simulink model "twoControllers"  (R2019b)
settings: Solver=VariableStepAuto  StartTime=0.0  StopTime=10.0  RelTol=1e-3
values from neighbouring files (symbols this model uses):
  g = 9.81    [G.m]    (also in connect_pend_runner.m = -9.81; run.m; single_pend_runner.m = -9.81)
  Kd = 50    [anujay_single_pendulum_same.m]    (also in connect_pend_runner.m = 10; double_pend_setup.m = [50,0;0,50]; run.m = 300; single_pend_runner.m = 500)
  Kp = 300    [run.m]    (also in single_pend_runner.m = 500)
  l = [ 1.0, 1.5]    [double_pend_setup.m]    (also in run.m = 2)
  m = 10    [run.m]
undefined symbols (not defined in the file or in its folder): Kd2, Kp2, T
libraries: robotcorelib x1
settings Model: Creator=nathanielgoldfarb  LastModifiedBy=nathanielgoldfarb

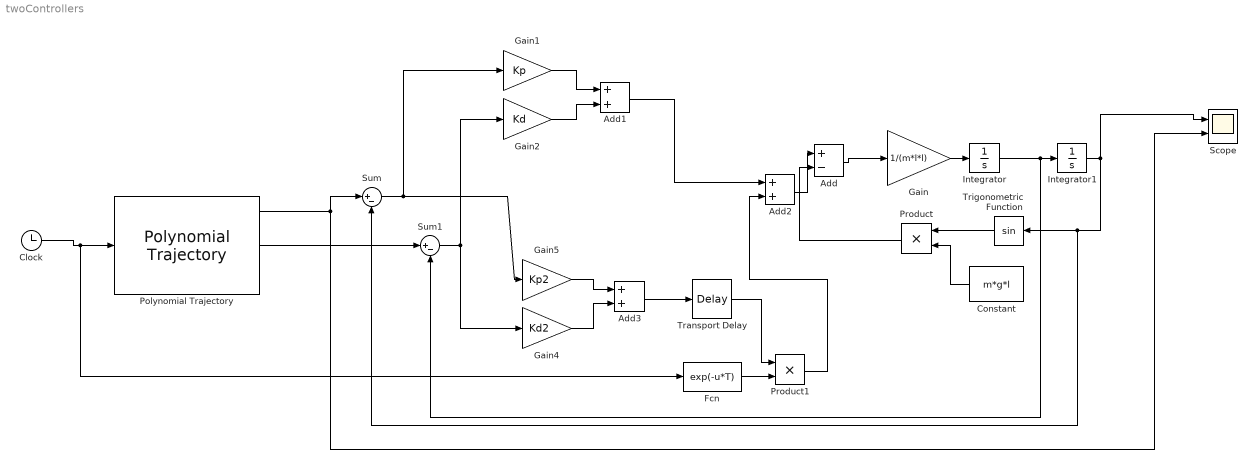
== system twoControllers ==
  Add : Sum  Inputs=+-
  Add1 : Sum
  Add2 : Sum
  Add3 : Sum
  Clock : Clock
  Constant : Constant  Value=m*g*l
  Fcn : Fcn  Expr=exp(-u*T)
  Gain : Gain  Gain=1/(m*l*l)
  Gain1 : Gain  Gain=Kp
  Gain2 : Gain  Gain=Kd
  Gain4 : Gain  Gain=Kd2
  Gain5 : Gain  Gain=Kp2
  Integrator : Integrator
  Integrator1 : Integrator  InitialCondition=-pi
  Polynomial Trajectory : robotcorelib/Polynomial Trajectory  WaypointSource=Internal  Waypoints=[ -pi , 0 ]  TimePoints=[ 0, 3]  TimeInterval=[ 1, 4 ]  Method=Cubic Polynomial  ParameterSource=Internal  VelocityBoundaryCondition=zeros( 1, 2 )  AccelerationBoundaryCondition=zeros( 2, 5 )  SimulateUsing=Interpreted execution
      settings: SourceProductName=Robotics System Toolbox  SourceProductBaseCode=RO
  Product : Product
  Product1 : Product
  Scope : Scope  NumInputPorts=2
  Sum : Sum  Inputs=|+-
  Sum1 : Sum  Inputs=|+-
  Transport Delay : TransportDelay  DelayTime=.1
  Trigonometric Function : Trigonometry
  wires:
  Trigonometric Function/1 -> Product/1
  Product/1 -> Add/2
  Integrator1/1 -> Scope/1, Trigonometric Function/1, Sum/2
  Polynomial Trajectory/1 -> Scope/2, Sum/1
  Polynomial Trajectory/2 -> Sum1/1
  Sum1/1 -> Gain4/1, Gain2/1
  Gain/1 -> Integrator/1
  Integrator/1 -> Sum1/2, Integrator1/1
  Add/1 -> Gain/1
  Clock/1 -> Fcn/1, Polynomial Trajectory/1
  Constant/1 -> Product/2
  Sum/1 -> Gain1/1, Gain5/1
  Gain5/1 -> Add3/1
  Gain4/1 -> Add3/2
  Gain2/1 -> Add1/2
  Gain1/1 -> Add1/1
  Add1/1 -> Add2/1
  Add3/1 -> Transport Delay/1
  Add2/1 -> Add/1
  Transport Delay/1 -> Product1/1
  Fcn/1 -> Product1/2
  Product1/1 -> Add2/2
